simulink model "Cowley_TakeHomeFinalSim"  (R2020b)
settings: Solver=VariableStepAuto  StartTime=0.0  StopTime=50  RelTol=1e-3
values from neighbouring files (symbols this model uses):
  c1 = 2.4    [Cowley_FinalTakeHome1.m]    (also in Cowley_FinalTakeHome234.m = 0; Cowley_FinalTakeHome5.m = 0)
  c2 = 0.3    [Cowley_FinalTakeHome1.m]    (also in Cowley_FinalTakeHome234.m = 0; Cowley_FinalTakeHome5.m = 0)
  F20 = 3    [Cowley_FinalTakeHome1.m]    (also in Cowley_FinalTakeHome234.m = 1; Cowley_FinalTakeHome5.m = 0)
  k1 = 10000    [Cowley_315Week13HW_Problem2.m]    (also in Cowley_FinalTakeHome1.m = 24; Cowley_FinalTakeHome234.m = 24; Cowley_FinalTakeHome5.m = 24)
  k2 = 20000    [Cowley_315Week13HW_Problem2.m]    (also in Cowley_FinalTakeHome1.m = 3; Cowley_FinalTakeHome234.m = 3; Cowley_FinalTakeHome5.m = 3)
  m1 = 75    [Cowley_315Week13HW_Problem2.m]    (also in Cowley_FinalTakeHome1.m = 9; Cowley_FinalTakeHome234.m = 9; Cowley_FinalTakeHome5.m = 9)
  m2 = 100    [Cowley_315Week13HW_Problem2.m]    (also in Cowley_FinalTakeHome1.m = 1; Cowley_FinalTakeHome234.m = 1; Cowley_FinalTakeHome5.m = 1)
  v10 = 1    [Cowley_FinalTakeHome1.m]    (also in Cowley_FinalTakeHome234.m = 0; Cowley_FinalTakeHome5.m = 0.111111111111)
  v20 = -1    [Cowley_FinalTakeHome1.m]    (also in Cowley_FinalTakeHome234.m = 0; Cowley_FinalTakeHome5.m = 0)
  w = 30    [Cowley_315Exam2TakeHome.m]    (also in Cowley_315Week8HW_Prob2.m = 10; Cowley_FinalTakeHome1.m = 1; Cowley_FinalTakeHome234.m = 2; Cowley_FinalTakeHome5.m = 0)
  x10 = 0.1    [Cowley_FinalTakeHome1.m]    (also in Cowley_FinalTakeHome234.m = 0; Cowley_FinalTakeHome5.m = 0)
  x20 = 0    [Cowley_FinalTakeHome1.m]    (also in Cowley_FinalTakeHome234.m; Cowley_FinalTakeHome5.m)
settings Model: Creator=mattcowley  LastModifiedBy=mattcowley

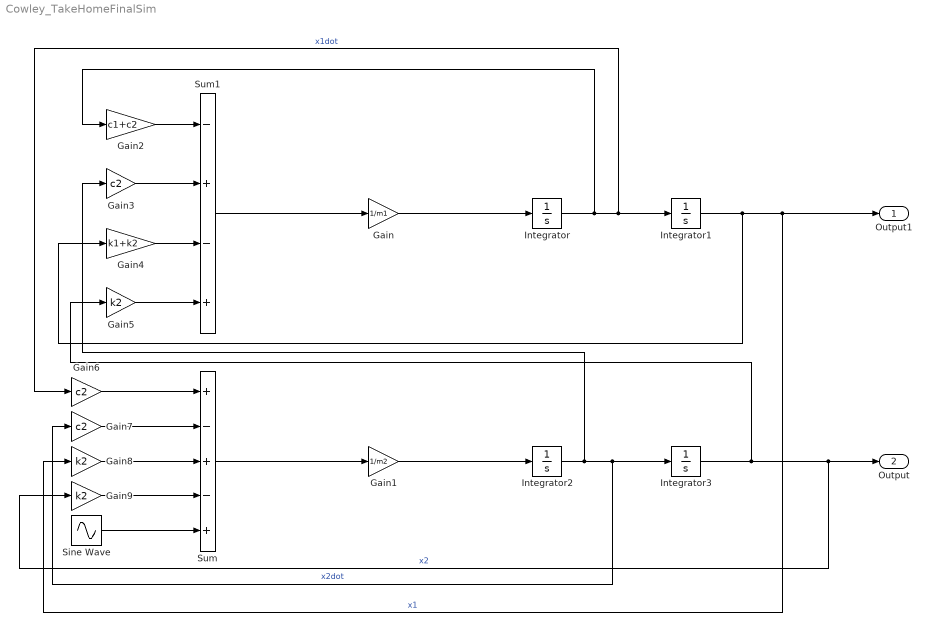
== system Cowley_TakeHomeFinalSim ==
  Gain : Gain  Gain=1/m1
  Gain1 : Gain  Gain=1/m2
  Gain2 : Gain  Gain=c1+c2
  Gain3 : Gain  Gain=c2
  Gain4 : Gain  Gain=k1+k2
  Gain5 : Gain  Gain=k2
  Gain6 : Gain  Gain=c2
  Gain7 : Gain  Gain=c2
  Gain8 : Gain  Gain=k2
  Gain9 : Gain  Gain=k2
  Integrator : Integrator  InitialCondition=v10
  Integrator1 : Integrator  InitialCondition=x10
  Integrator2 : Integrator  InitialCondition=v20
  Integrator3 : Integrator  InitialCondition=x20
  Sine Wave : Sin  Amplitude=F20  Frequency=w  Phase=pi/2  SampleTime=0
  Sum : Sum  Inputs=+-+-+
  Sum1 : Sum  Inputs=-+-+
  Output1 : Outport  SignalName=x1
  Output : Outport  Port=2  SignalName=x2
  wires:
  Sine Wave/1 -> Sum/5
  Gain1/1 -> Integrator2/1
  Integrator2/1 -> Gain3/1, Gain7/1, Integrator3/1  "x2dot"
  Integrator1/1 -> Gain4/1, Gain8/1, Output1/1  "x1"
  Integrator3/1 -> Gain5/1, Gain9/1, Output/1  "x2"
  Sum1/1 -> Gain/1
  Gain/1 -> Integrator/1
  Integrator/1 -> Gain2/1, Gain6/1, Integrator1/1  "x1dot"
  Sum/1 -> Gain1/1
  Gain5/1 -> Sum1/4
  Gain4/1 -> Sum1/3
  Gain3/1 -> Sum1/2
  Gain2/1 -> Sum1/1
  Gain9/1 -> Sum/4
  Gain8/1 -> Sum/3
  Gain7/1 -> Sum/2
  Gain6/1 -> Sum/1
